simulink model "Mockup_Gestures"  (R2018b)
settings: Solver=VariableStepAuto  StartTime=0.0  StopTime=10.0  RelTol=1e-3
undefined symbols (not defined in the file or in its folder): serial
libraries: instrumentlib x2, dspstat3 x1, dspnetwork x1
settings Model: Creator=anton  LastModifiedBy=anton

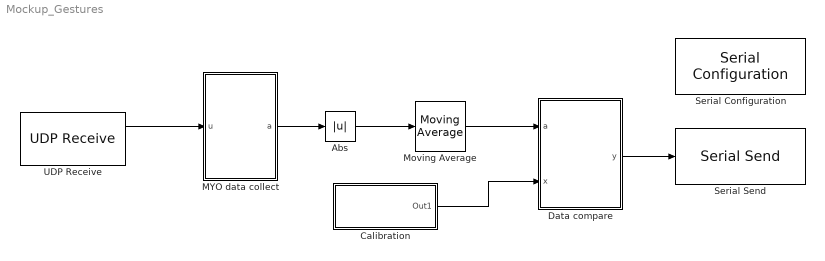
== system Mockup_Gestures ==
  Abs : Abs
  "Calibration " : Subsystem
  "Data compare " : MATLAB Function  TreatAsAtomicUnit=on
  "MYO data collect " : MATLAB Function  TreatAsAtomicUnit=on
  Moving Average : dspstat3/Moving Average  Method=Sliding window  ForgettingFactorPort=off  SpecifyWindowLength=on  WindowLength=50  ForgettingFactor=0.9  SimulateUsing=Code generation
  Serial Configuration : instrumentlib/Serial Configuration  Priority=-200000  ComPortMenu=<Please select a port...>  ComPort=COM5  ObjConstructor=serial('COM5');  BaudRate=9600  DataBits=8  Parity=none  StopBits=1  FlowControl=none  Timeout=10  ByteOrder=LittleEndian
  Serial Send : instrumentlib/Serial Send  ComPortMenu=<Please select a port...>  ComPort=COM5  ObjConstructor=serial('COM5');  Terminator=<none>  EnableBlockingMode=on
  UDP Receive : dspnetwork/UDP Receive  localURL='0.0.0.0'  localPort=54000  remoteURL='0.0.0.0'  remotePort=-1  recvBufferSize=32  dims=255  signalDatatype=int8  isVarSize=off  showBlockingTime=off  blockingTime=0  sampletime=0.02  blockPlatform=[]
      settings: SourceProductName=DSP System Toolbox  SourceProductBaseCode=DS
  wires:
  "Calibration "/1(Out1) -> "Data compare "/2(x)
  Moving Average/1 -> "Data compare "/1(a)
  "MYO data collect "/1(a) -> Abs/1
  "Data compare "/1(y) -> Serial Send/1
  Abs/1 -> Moving Average/1
  UDP Receive/1 -> "MYO data collect "/1(u)

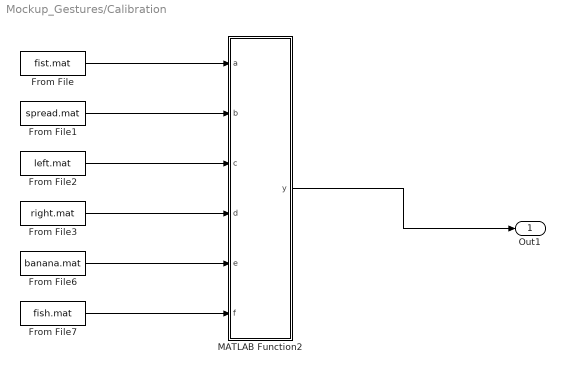
== system Mockup_Gestures/Calibration  ==
  From File : FromFile  FileName=fist.mat  OutDataTypeStr=double  SampleTime=0  ExtrapolationBeforeFirstDataPoint=Hold first value  InterpolationWithinTimeRange=Zero order hold  ExtrapolationAfterLastDataPoint=Hold last value
  From File1 : FromFile  FileName=spread.mat  OutDataTypeStr=double  SampleTime=0  ExtrapolationBeforeFirstDataPoint=Hold first value  InterpolationWithinTimeRange=Zero order hold  ExtrapolationAfterLastDataPoint=Hold last value
  From File2 : FromFile  FileName=left.mat  OutDataTypeStr=double  SampleTime=0  ExtrapolationBeforeFirstDataPoint=Hold first value  InterpolationWithinTimeRange=Zero order hold  ExtrapolationAfterLastDataPoint=Hold last value
  From File3 : FromFile  FileName=right.mat  OutDataTypeStr=double  SampleTime=0  ExtrapolationBeforeFirstDataPoint=Hold first value  InterpolationWithinTimeRange=Zero order hold  ExtrapolationAfterLastDataPoint=Hold last value
  From File6 : FromFile  FileName=banana.mat  OutDataTypeStr=double  SampleTime=0  ExtrapolationBeforeFirstDataPoint=Hold first value  InterpolationWithinTimeRange=Zero order hold  ExtrapolationAfterLastDataPoint=Hold last value
  From File7 : FromFile  FileName=fish.mat  OutDataTypeStr=double  SampleTime=0  ExtrapolationBeforeFirstDataPoint=Hold first value  InterpolationWithinTimeRange=Zero order hold  ExtrapolationAfterLastDataPoint=Hold last value
  MATLAB Function2 : MATLAB Function  TreatAsAtomicUnit=on
  Out1 : Outport
  wires:
  MATLAB Function2/1(y) -> Out1/1
  From File/1 -> MATLAB Function2/1(a)
  From File6/1 -> MATLAB Function2/5(e)
  From File1/1 -> MATLAB Function2/2(b)
  From File7/1 -> MATLAB Function2/6(f)
  From File3/1 -> MATLAB Function2/4(d)
  From File2/1 -> MATLAB Function2/3(c)

== matlab function Mockup_Gestures/Data compare  ==
  data: a input; y output; x input
function y  = fcn(a,x)

%Percentage
t = 1.6; %top
v = 0.55; %bot

%constant
n = 1;  %top
m = 1;  %bot

    if a<x(1,1)*t+n & a>x(2,1)*v-m & b<x(3,1)*t+n & b>x(4,1)*v-m & c<x(5,1)*t+n & c>x(6,1)*v-m & d<x(7,1)*t+n & d>x(8,1)*v-m & e<x(9,1)*t+n & e>x(10,1)*v-m & f<x(11,1)*t+n & f>x(12,1)*v-m & g<x(13,1)*t+n & g>x(14,1)*v-m & h<x(15,1)*t+n & h>x(16,1)*v-m 
        y=1;
    elseif a<x(1,2)*t+n & a>x(2,2)*v-m & b<x(3,2)*t+n & b>x(4,2)*v-m & c<x(5,2)*t+n & c>x(6,2)*v-m & d<x(7,2)*t+n & d>x(8,2)*v-m & e<x(9,2)*t+n & e>x(10,2)*v-m & f<x(11,2)*t+n & f>x(12,2)*v-m & g<x(13,2)*t+n & g>x(14,2)*v-m & h<x(15,2)*t+n & h>x(16,2)*v-m 
        y=2;
    elseif a<x(1,3)*t+n & a>x(2,3)*v-m & b<x(3,3)*t+n & b>x(4,3)*v-m & c<x(5,3)*t+n & c>x(6,3)*v-m & d<x(7,3)*t+n & d>x(8,3)*v-m & e<x(9,3)*t+n & e>x(10,3)*v-m & f<x(11,3)*t+n & f>x(12,3)*v-m & g<x(13,3)*t+n & g>x(14,3)*v-m & h<x(15,3)*t+n & h>x(16,3)*v-m 
        y=3;
    elseif a<x(1,4)*t+n & a>x(2,4)*v-m & b<x(3,4)*t+n & b>x(4,4)*v-m & c<x(5,4)*t+n & c>x(6,4)*v-m & d<x(7,4)*t+n & d>x(8,4)*v-m & e<x(9,4)*t+n & e>x(10,4)*v-m & f<x(11,4)*t+n & f>x(12,4)*v-m & g<x(13,4)*t+n & g>x(14,4)*v-m & h<x(15,4)*t+n & h>x(16,4)*v-m 
        y=4;
    elseif a<x(1,5)*t+n & a>x(2,5)*v-m & b<x(3,5)*t+n & b>x(4,5)*v-m & c<x(5,5)*t+n & c>x(6,5)*v-m & d<x(7,5)*t+n & d>x(8,5)*v-m & e<x(9,5)*t+n & e>x(10,5)*v-m & f<x(11,5)*t+n & f>x(12,5)*v-m & g<x(13,5)*t+n & g>x(14,5)*v-m & h<x(15,5)*t+n & h>x(16,5)*v-m 
        y=5;
    elseif a<x(1,6)*t+n & a>x(2,6)*v-m & b<x(3,6)*t+n & b>x(4,6)*v-m & c<x(5,6)*t+n & c>x(6,6)*v-m & d<x(7,6)*t+n & d>x(8,6)*v-m & e<x(9,6)*t+n & e>x(10,6)*v-m & f<x(11,6)*t+n & f>x(12,6)*v-m & g<x(13,6)*t+n & g>x(14,6)*v-m & h<x(15,6)*t+n & h>x(16,6)*v-m 
        y=6;
               
    else
y=0
    
    end

% %Threshold with Addition
% t = 9;
% v = 3;
% 
%     if a<x(1,1)+t & a>x(2,1)-v & b<x(3,1)+t & b>x(4,1)-v & c<x(5,1)+t & c>x(6,1)-v & d<x(7,1)+t & d>x(8,1)-v & e<x(9,1)+t & e>x(10,1)-v & f<x(11,1)+t & f>x(12,1)-v & g<x(13,1)+t & g>x(14,1)-v & h<x(15,1)+t & h>x(16,1)-v 
%         y=1;
%     elseif a<x(1,2)+t & a>x(2,2)-v & b<x(3,2)+t & b>x(4,2)-v & c<x(5,2)+t & c>x(6,2)-v & d<x(7,2)+t & d>x(8,2)-v & e<x(9,2)+t & e>x(10,2)-v & f<x(11,2)+t & f>x(12,2)-v & g<x(13,2)+t & g>x(14,2)-v & h<x(15,2)+t & h>x(16,2)-v 
%         y=2;
%     elseif a<x(1,3)+t & a>x(2,3)-v & b<x(3,3)+t & b>x(4,3)-v & c<x(5,3)+t & c>x(6,3)-v & d<x(7,3)+t & d>x(8,3)-v & e<x(9,3)+t & e>x(10,3)-v & f<x(11,3)+t & f>x(12,3)-v & g<x(13,3)+t & g>x(14,3)-v & h<x(15,3)+t & h>x(16,3)-v 
%         y=3;
%     elseif a<x(1,4)+t & a>x(2,4)-v & b<x(3,4)+t & b>x(4,4)-v & c<x(5,4)+t & c>x(6,4)-v & d<x(7,4)+t & d>x(8,4)-v & e<x(9,4)+t & e>x(10,4)-v & f<x(11,4)+t & f>x(12,4)-v & g<x(13,4)+t & g>x(14,4)-v & h<x(15,4)+t & h>x(16,4)-v 
%         y=4;
%     elseif a<x(1,5)+t & a>x(2,5)-v & b<x(3,5)+t & b>x(4,5)-v & c<x(5,5)+t & c>x(6,5)-v & d<x(7,5)+t & d>x(8,5)-v & e<x(9,5)+t & e>x(10,5)-v & f<x(11,5)+t & f>x(12,5)-v & g<x(13,5)+t & g>x(14,5)-v & h<x(15,5)+t & h>x(16,5)-v 
%         y=5;
%     elseif a<x(1,6)+t & a>x(2,6)-v & b<x(3,6)+t & b>x(4,6)-v & c<x(5,6)+t & c>x(6,6)-v & d<x(7,6)+t & d>x(8,6)-v & e<x(9,6)+t & e>x(10,6)-v & f<x(11,6)+t & f>x(12,6)-v & g<x(13,6)+t & g>x(14,6)-v & h<x(15,6)+t & h>x(16,6)-v 
%         y=6;
%     elseif a<x(1,7)+t & a>x(2,7)-v & b<x(3,7)+t & b>x(4,7)-v & c<x(5,7)+t & c>x(6,7)-v & d<x(7,7)+t & d>x(8,7)-v & e<x(9,7)+t & e>x(10,7)-v & f<x(11,7)+t & f>x(12,7)-v & g<x(13,7)+t & g>x(14,7)-v & h<x(15,7)+t & h>x(16,7)-v 
%         y=7;
%     elseif a<x(1,8)+t & a>x(2,8)-v & b<x(3,8)+t & b>x(4,8)-v & c<x(5,8)+t & c>x(6,8)-v & d<x(7,8)+t & d>x(8,8)-v & e<x(9,8)+t & e>x(10,8)-v & f<x(11,8)+t & f>x(12,8)-v & g<x(13,8)+t & g>x(14,8)-v & h<x(15,8)+t & h>x(16,8)-v 
%         y=8;
%             
%     else
% y=0
%     
%     end

== matlab function Mockup_Gestures/MYO data collect  ==
  data: u input; a output
%a is the output of this block, and fcn(u) is the input required
function a   = fcn(u)
        
%Below the output a is specified as the 3 row of the 8x1 input vector u
a = u(1,:);
b = u(2,:);
c = u(3,:);
d = u(4,:);
e = u(5,:);
f = u(6,:);
g = u(7,:);
h = u(8,:);

== matlab function Mockup_Gestures/Calibration /MATLAB Function2 ==
  data: a input; b input; c input; d input; e input; f input; y output
function y = fcn(a, b, c, d, e, f)

y=[a b c d e f];
